simulink model "CD2_Infiltration_v01"  (Simulink 6.4)
settings: Solver=FixedStepDiscrete  StartTime=0  StopTime=12000  FixedStep=300  RelTol=1e-3
undefined symbols (not defined in the file or in its folder): table, tablestep
settings Model: LastModifiedBy=c81523
settings DataIOCC: LimitDataPoints=off  TimeSaveName=cd_time  SignalLoggingName=sigsOut
settings DebuggingCC: SolverPrmCheckMsg=none  StrictBusMsg=None
settings HardwareCC: TargetUnknown=on

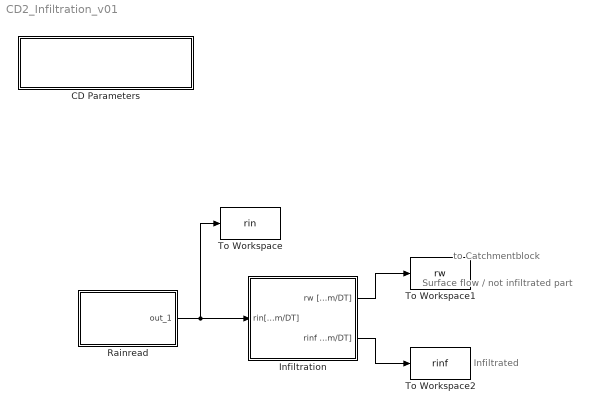
== system CD2_Infiltration_v01 ==
  note: to Catchmentblock
  note: Infiltrated
  note: Surface flow / not infiltrated part
  CD Parameters : Subsystem  mask(City Drain 1.0 - Simulation parameters ){t_step=300, t_start=0, t_stop=12000}
      mask prompts: t_step "Sampling Time [s]"; t_start "Start Time [s]"; t_stop "Stop Time [s]"
      mask help:
      | Block that sets the global parameters required in City Drain 1.0. Following paramters are set without user's input:
      |
      | - 'Solver' --> 'FixedStepDiscrete'
      | - 'TimeSaveName' --> 'cd_time'
      | - 'Decimation' --> '1'
      | - 'LimitDataPoints' -->  'off'
      mask init:
      | % toplevel systems' name --> Plant file name;
      | tls=bdroot(gcb); 
      | set_param(tls, 'Solver', 'FixedStepDiscrete'); 
      | set_param(tls, 'TimeSaveName', 'cd_time');
      | set_param(tls, 'Decimation', '1');
      | set_param(tls, 'LimitDataPoints', 'off');
      | set_param(tls, 'ScreenColor', 'white');
      | 
      | tstep_char=num2str(t_step); % Setting the discrete time step
      | set_param(tls, 'FixedStep', tstep_char); 
      | 
      | tstart_char=num2str(t_start); % Setting the start time
      | set_param(tls, 'StartTime', tstart_char); 
      | 
      | tstop_char=num2str(t_stop); % Setting the stop time
      | set_param(tls, 'StopTime', tstop_char);
      mask Display:
      | plot(0,0,100,100);
      | 
      | text(50,65,'CITY DRAIN','HorizontalAlignment','center');
      | text(50,35,'PARAMETERS','HorizontalAlignment','center');
      | 
      | 
      | image(imread('CityDrain_SimParam.jpg'))
  Infiltration : Subsystem  mask(ATV 138 - Dynamic Infiltration){Ared=100, phiinf=0.2, kf=0.00005, Rsu=0.1, rDn=131.7, D=30, fz=1.2}
      mask prompts: Ared "Ared [ha] - Reduced (flow contributing areas"; phiinf "phi [ - ] - Portion of infiltrated area Ared/(Au+As)"; kf "kf [m/s] - permiability of swale's soil material"; Rsu "As/Au [ 0.1 - 0.2 ] - Ratio of swale area (As) to connected Area (Au)"; rDn "rD(n) [l/(s.ha)] - Design rain intensity of the swale"; D "D [min] - Duration of design rain rD(n)"; fz "fz [-] - Loading coefficient (ATV A117)"
      mask help:
      | Infiltration block
      | Dynamic swale infiltration according to ATV 138. Infiltration rates and swale volume is design according to ATV 138.
      | Block used r[mm/DT] as input and output. Thus the block is designed as "pre-block" to catchment type blocks entering at rain input.
      |
      | Function used:
      | No other specific functions used than standard city drain functions.
      mask init:
      | % reading the toplevel systems' name 
      | % --> Plant file name;
      | tls=bdroot(gcb); 
      | % Obtaining the fixed sampling time
      | t_samp_char=get_param(tls, 'FixedStep');
      | % Convertion to numeric value
      | tstep = str2num(t_samp_char); 
      | 
      | % Calculations for Infiltration
      | Asu=Ared.*phiinf; 	% in [ha]
      | 
      | Au=Asu./(1+Rsu); 	% in [ha]
      | As=Asu-Au;			% in [ha]
      | 
      | qs=As.*10000.*kf./2; % [m3/s]
      | V=((Au+As).*10000.*10.^(-7).*rDn-qs).*D.*60.*fz; % [m3]
      mask Display:
      | plot(0,0,100,100);
      | 
      | 
      | text(50,60,'INF','HorizontalAlignment','center');
      | text(50,40,'ATV','HorizontalAlignment','center');
      | text(50,20,'138','HorizontalAlignment','center');
      | 
      | port_label('input',1,'rin');
      | port_label('output',1,'rw');
      | port_label('output',2,'rinf');
  Rainread : Subsystem  mask(Rain Read){table0='test2.km2', crep=off}
      mask prompts: table0 "Filename"; crep "Cylic repitition"
      mask help:
      | Read raindata from ASCII File in following formats:
      |
      | *.ixx ... Format used by the Austrian Hydrographic Service.
      | *.km2 ... Format used in the Mouse Software from DHI (Danish Hydraulic Institute)
      | *.mse ... modified mse format used in  Mouse Software from DHI (Danish Hydraulic Institute)
      |
      | Used function: CD1_mfun_rainread.m
      mask init:
      | % cache table size set to 1000
      | %table=zeros(1000,2)
      | [table,tablestep]=CD1_mfun_rainread(table0);
      | 
      | % reading the toplevel systems' name 
      | % --> Plant file name;
      | tls=bdroot(gcb); 
      | % Obtaining the fixed sampling time
      | t_samp_char=get_param(tls, 'FixedStep');
      | % Convertion to numeric value
      | tstep = str2num(t_samp_char);
      mask Display:
      | plot(0,0,100,100);
      | 
      | text(40,40,'RAIN READ');
      | plot(
      | [5 10 10 15 15 20 20 25 25 30 30 40 40 45],
      | [0 0 20 20 40 40 60 60 30 30 0 0 0 0]+20);
  To Workspace : ToWorkspace  VariableName=rin  SampleTime=-1  SaveFormat=Array
  To Workspace1 : ToWorkspace  VariableName=rw  SampleTime=-1  SaveFormat=Array
  To Workspace2 : ToWorkspace  VariableName=rinf  SampleTime=-1  SaveFormat=Array
  wires:
  Infiltration/1(rw [mm/DT]) -> To Workspace1/1
  Infiltration/2(rinf [mm/DT]) -> To Workspace2/1
  Rainread/1(out_1) -> Infiltration/1(rin[mm/DT]), To Workspace/1

== system CD2_Infiltration_v01/CD Parameters ==

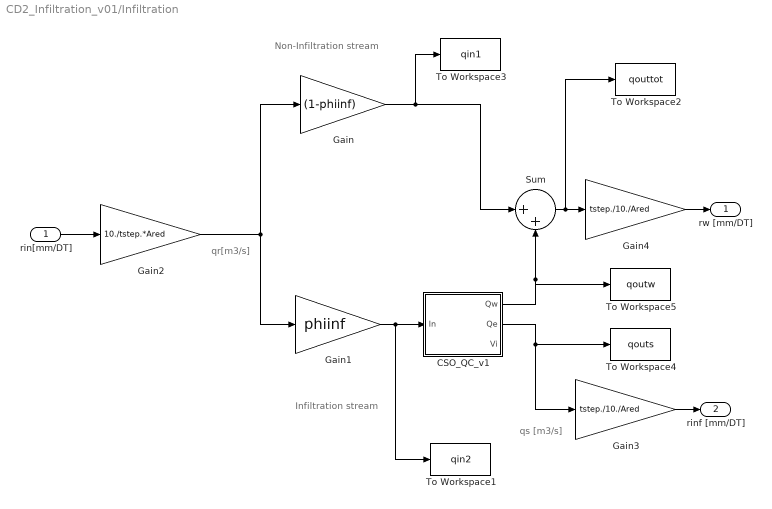
== system CD2_Infiltration_v01/Infiltration ==
  note: qr[m3/s]
  note: Infiltration stream
  note: Non-Infiltration stream
  note: qs [m3/s]
  rin[mm/DT] : Inport
  CSO_QC_v1 : Subsystem  mask(CSO Typ B - Combined sewer overflow){Vmax=V, Qemax=qs, n_comp=0, n_sed=[]}
      mask prompts: Vmax "Basin Volume (m3)"; Qemax "Maximum Effluent flow [m3/s]"; n_comp "Number of Pollutants [-]"; n_sed "n-sed (Vect. of Sed. Coefficients)"
      mask help:
      | Combined sewer overflow structure.
      | Diverts the inflow given into effluent and overflow. The model implemented consideres hydraulics and pollutant routing by full mixing in the structure.
      |
      | In addition to Type A a retenetion/sedimentation factor is introduced. The factor may be used for applying different ratios in pollutant concentration for effluent flow (QE) and overflow (QW).
      |
      | Function used:
      | CD1_sfun_cso_B.m
      mask init:
      | % reading the toplevel systems' name 
      | % --> Plant file name;
      | tls=bdroot(gcb); 
      | % Obtaining the fixed sampling time
      | t_samp_char=get_param(tls, 'FixedStep');
      | % Convertion to numeric value
      | tstep = str2num(t_samp_char);
      mask Display:
      | plot(0,0,100,100);
      | 
      | 
      | text(50,60,'CSO','HorizontalAlignment','center');
      | text(50,30,'Typ B','HorizontalAlignment','center');
      | 
      | 
      | port_label('input',1,'Qi');
      | port_label('output',1,'Qw');
      | port_label('output',2,'Qe');
      | port_label('output',3,'Vi');
  Gain : Gain  Gain=(1-phiinf)  SaturateOnIntegerOverflow=on
  Gain1 : Gain  Gain=phiinf  SaturateOnIntegerOverflow=on
  Gain2 : Gain  Gain=10./tstep.*Ared  SaturateOnIntegerOverflow=on
  Gain3 : Gain  Gain=tstep./10./Ared  SaturateOnIntegerOverflow=on
  Gain4 : Gain  Gain=tstep./10./Ared  SaturateOnIntegerOverflow=on
  Sum : Sum  Inputs=|++  SaturateOnIntegerOverflow=on
  To Workspace1 : ToWorkspace  VariableName=qin2  SampleTime=-1  SaveFormat=Array
  To Workspace2 : ToWorkspace  VariableName=qouttot  SampleTime=-1  SaveFormat=Array
  To Workspace3 : ToWorkspace  VariableName=qin1  SampleTime=-1  SaveFormat=Array
  To Workspace4 : ToWorkspace  VariableName=qouts  SampleTime=-1  SaveFormat=Array
  To Workspace5 : ToWorkspace  VariableName=qoutw  SampleTime=-1  SaveFormat=Array
  rw [mm/DT] : Outport
  rinf [mm/DT] : Outport  Port=2
  wires:
  rin[mm/DT]/1 -> Gain2/1
  Gain2/1 -> Gain1/1, Gain/1
  Gain1/1 -> CSO_QC_v1/1(In), To Workspace1/1
  Gain3/1 -> rinf [mm/DT]/1
  CSO_QC_v1/2(Qe) -> Gain3/1, To Workspace4/1
  CSO_QC_v1/1(Qw) -> Sum/2, To Workspace5/1
  Gain/1 -> Sum/1, To Workspace3/1
  Sum/1 -> Gain4/1, To Workspace2/1
  Gain4/1 -> rw [mm/DT]/1

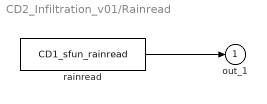
== system CD2_Infiltration_v01/Rainread ==
  rainread : S-Function  FunctionName=CD1_sfun_rainread  Parameters=crep,table,tablestep,tstep
  out_1 : Outport
  wires:
  rainread/1 -> out_1/1

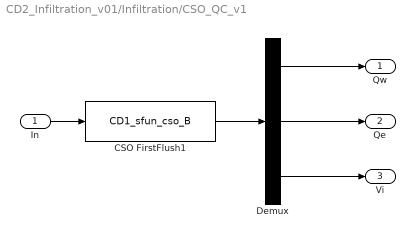
== system CD2_Infiltration_v01/Infiltration/CSO_QC_v1 ==
  In : Inport
  CSO FirstFlush1 : S-Function  FunctionName=CD1_sfun_cso_B  Parameters=Vmax,Qemax,n_comp,n_sed,tstep
  Demux : Demux  Outputs=[ (n_comp+1) (n_comp+1) (n_comp+1)]
  Qw : Outport
  Qe : Outport  Port=2
  Vi : Outport  Port=3
  wires:
  In/1 -> CSO FirstFlush1/1
  CSO FirstFlush1/1 -> Demux/1
  Demux/1 -> Qw/1
  Demux/2 -> Qe/1
  Demux/3 -> Vi/1
